simulink model "BMSBalancingLogic"  (R2025a)
settings: configuration reference "VehicleFixed5s" (kept outside this file)
model workspace (MAT data in the model file):
  BalNotActWait = 30
  BalOffWait = 20
  BalOnWait = 60
  TargetDeltaV = 0.00999999977648
  flgEnBalancing = 1
undefined symbols (not defined in the file): PlntBattNumCellSer
settings Model: DataDictionary=VirtualVehicleTemplate.sldd  ModifiedByFormat=The MathWorks, Inc.  ExtModeTrigDuration=5  Creator=The MathWorks, Inc.  LastModifiedBy=The MathWorks, Inc.
settings ConfigSetRef: SourceName=VehicleFixed5s

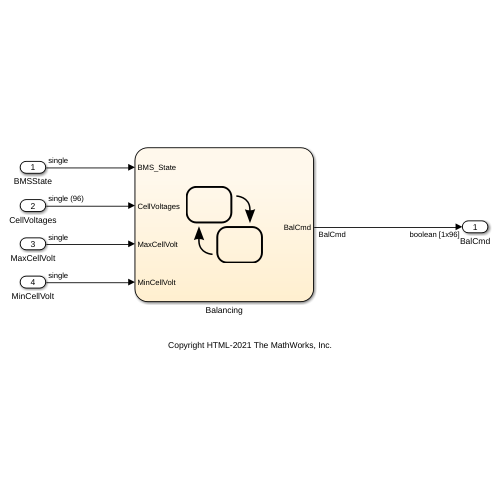
[thumbnail: Simulink's stored preview of the top-level diagram]
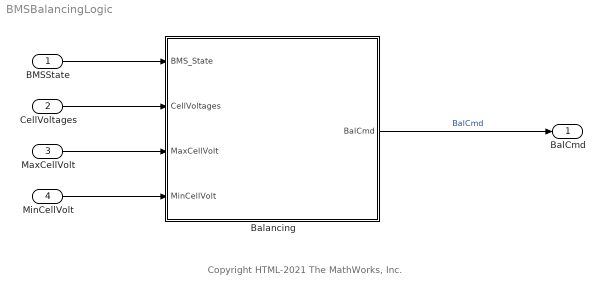
== system BMSBalancingLogic ==
  note: Copyright HTML-2021 The MathWorks, Inc.
  BMSState : Inport  OutDataTypeStr=single  PortDimensions=1  SampleTime=[5,0]
  CellVoltages : Inport  Port=2  OutDataTypeStr=single  PortDimensions=PlntBattNumCellSer  SampleTime=[5,0]
  MaxCellVolt : Inport  Port=3  OutDataTypeStr=single
  MinCellVolt : Inport  Port=4  OutDataTypeStr=single
  Balancing : Stateflow chart  TreatAsAtomicUnit=on  VariantControl=(default)
  BalCmd : Outport  OutDataTypeStr=boolean  PortDimensions=[1, PlntBattNumCellSer]  SampleTime=[5,0]  VectorParamsAs1DForOutWhenUnconnected=off
  wires:
  MinCellVolt/1 -> Balancing/4(MinCellVolt)
  MaxCellVolt/1 -> Balancing/3(MaxCellVolt)
  CellVoltages/1 -> Balancing/2(CellVoltages)
  Balancing/1(BalCmd) -> BalCmd/1  "BalCmd"
  BMSState/1 -> Balancing/1(BMS_State)

== stateflow chart BMSBalancingLogic/Balancing ==
  state BalancingOFF
    en:
    BalCmd(:,:) = false;
    en,du:
    DeltaCellVolt = MaxCellVolt - MinCellVolt;
  state BalancingON
    en, du:
    DeltaCellVolt = MaxCellVolt - MinCellVolt;
    state BalActive
      en, du:
      BalCmd = ((CellVoltages - MinCellVolt) > TargetDeltaV/2)';
      flgBalCompl = all(~BalCmd);
    state BalNotActive
    (default) -> BalActive
    BalNotActive -> BalActive [order 1] : [after(BalNotActWait,sec) && ...
        | DeltaCellVolt > TargetDeltaV]
    BalActive -> BalNotActive : [flgBalCompl]
  (default) -> BalancingOFF : {flgBalCompl = true;}
  BalancingOFF -> BalancingON : [flgEnBalancing && ...
      | BMS_State ~= 2 && ...
      | after(BalOffWait,sec) && ...
      | DeltaCellVolt > TargetDeltaV]
  BalancingON -> BalancingOFF : [BMS_State == 2]
      | %In Driving State
  BalNotActive -> BalancingOFF [order 2] : [after(BalOnWait,sec)]
  data: BMS_State input; CellVoltages input single; TargetDeltaV parameter; BalCmd output boolean size=[1, PlntBattNumCellSer] =boolean(zeros(1, PlntBattNumCellSer)); flgBalCompl local; MaxCellVolt input single; MinCellVolt input single; BalNotActWait parameter; BalOffWait parameter; BalOnWait parameter; flgEnBalancing parameter; DeltaCellVolt local single =single(0)
